simulink model "a2_2_g"  (R2023b)
settings: Solver=VariableStepAuto  StartTime=0.0  StopTime=10  RelTol=1e-3
settings Model: Creator=serkan  LastModifiedBy=serkan

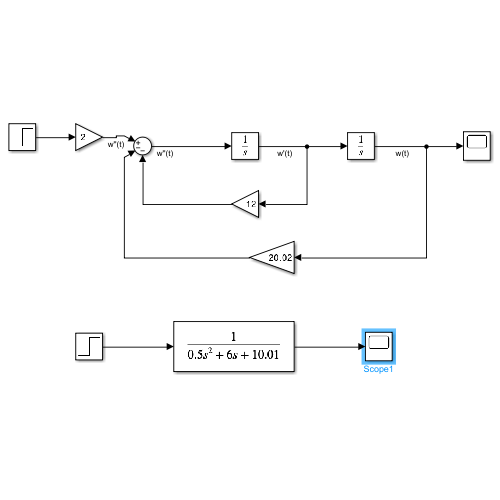
[thumbnail: Simulink's stored preview of the top-level diagram]
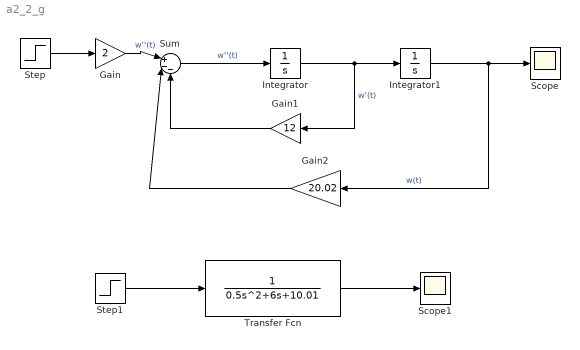
== system a2_2_g ==
  Gain : Gain  Gain=2
  Gain1 : Gain  Gain=12
  Gain2 : Gain  Gain=20.02
  Integrator : Integrator
  Integrator1 : Integrator
  Scope : Scope
  Scope1 : Scope
  Step : Step  SampleTime=0
  Step1 : Step  SampleTime=0
  Sum : Sum  Inputs=|+--
  Transfer Fcn : TransferFcn  Denominator=[0.5 6 10.01]
  wires:
  Integrator/1 -> Gain1/1, Integrator1/1  "w'(t)"
  Integrator1/1 -> Scope/1, Gain2/1  "w(t)"
  Sum/1 -> Integrator/1  "w''(t)"
  Step/1 -> Gain/1
  Gain/1 -> Sum/1  "w''(t)"
  Gain1/1 -> Sum/3
  Gain2/1 -> Sum/2
  Step1/1 -> Transfer Fcn/1
  Transfer Fcn/1 -> Scope1/1
